simulink model "abs_complex_test"  (Simulink 8.4)
settings: Solver=FixedStepDiscrete  StartTime=0.0  StopTime=10.0  FixedStep=1.0  RelTol=1e-3
settings Model: Creator=arnaud  LastModifiedBy=arnaud
settings DataIOCC: SaveFormat=Structure

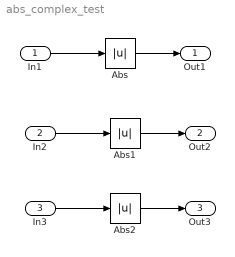
== system abs_complex_test ==
  In1 : Inport  OutDataTypeStr=double
      settings: SignalType=complex
  In2 : Inport  Port=2  OutDataTypeStr=double  PortDimensions=[3]
      settings: SignalType=complex
  In3 : Inport  Port=3  PortDimensions=[4 2]
      settings: SignalType=complex
  Abs : Abs
  Abs1 : Abs
  Abs2 : Abs
  Out1 : Outport
  Out2 : Outport  Port=2
  Out3 : Outport  Port=3
  wires:
  In1/1 -> Abs/1
  Abs/1 -> Out1/1
  In2/1 -> Abs1/1
  Abs1/1 -> Out2/1
  In3/1 -> Abs2/1
  Abs2/1 -> Out3/1
